simulink model "Minh_Final_project_Inverter_V3"  (R2024b)
settings: Solver=VariableStepAuto  StartTime=0.0  StopTime=100  FixedStep=1e-5  MaxStep=1e-3  MinStep=1e-8  RelTol=1e-2
values from neighbouring files (symbols this model uses):
  A_f = 1.24    [Minh_Inverter_Init.m]
  C_d = 0.7041    [Minh_Inverter_Init.m]
  C_rr = 0.02    [Minh_Inverter_Init.m]
  Current_max = min(InvCurr,mCurr)    [Minh_Inverter_Init.m]
  Encoder_Offset = (PhaseA_offset/ppair)*pi/180    (= -0.785398163397)    [Minh_Inverter_Init.m]
  g = 9.8    [Minh_Inverter_Init.m]
  J = mrot*r^2/k^2 + 0.0045    (= 0.8303048)    [Minh_Inverter_Init.m]
  k = 1    [Minh_Inverter_Init.m]
  lambda = 0.0375    [Minh_Inverter_Init.m]
  Ld = 0.1e-3    (= 0.0001)    [Minh_Inverter_Init.m]
  Lq = Ld    (= 0.0001)    [Minh_Inverter_Init.m]
  m = 1    [Minh_Inverter_Init.m]
  ppair = 4    [Minh_Inverter_Init.m]
  r = 0.4064/2    (= 0.2032)    [Minh_Inverter_Init.m]
  rho = 1.2    [Minh_Inverter_Init.m]
  Rs = (Rpp^2)/(Rpp*3)    (= 0.00433333333333)    [Minh_Inverter_Init.m]
  speed_max = rpm_max*2*pi/60    (= 523.598775598)    [Minh_Inverter_Init.m]
  Torque_max = Current_max*3*lambda*ppair/2    [Minh_Inverter_Init.m]
  Voltage_max = min(V_bat,mVolt)    [Minh_Inverter_Init.m]
undefined symbols (not defined in the file or in its folder): Down, Up
libraries: nesl_utility x27, fl_lib x23, slpidlib x12, ee_lib x11, spsabctodq0Lib x4, simulink x3, spsdq0toabcLib x2, eePwmGenerator x2, mcbresolverdecoderlib x1, eeResolverToDigitalConverter x1
(part 2 of 3)

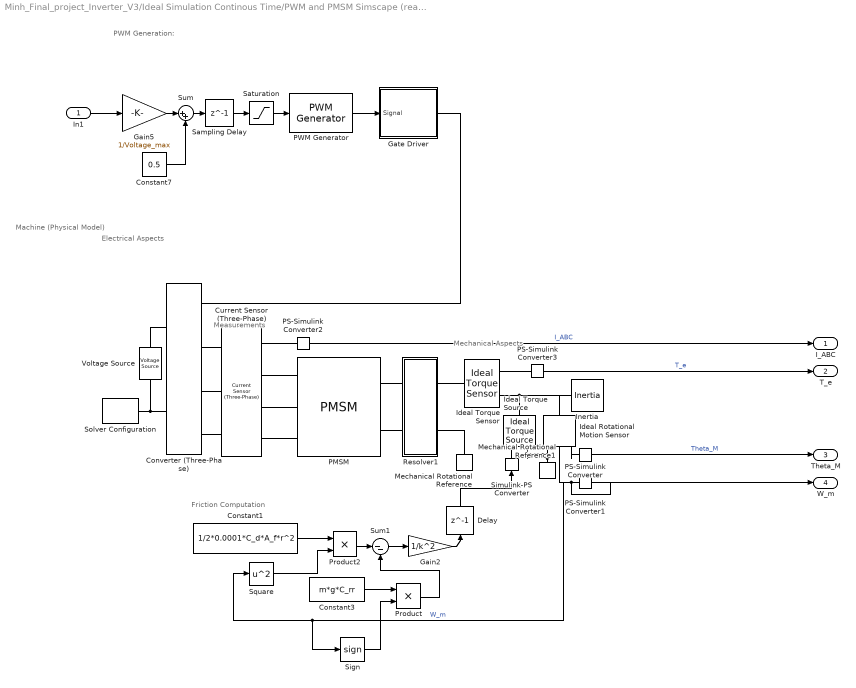
== system Minh_Final_project_Inverter_V3/Ideal Simulation Continous Time/PWM and PMSM Simscape (real model) ==
  note: Friction Computation
  note: Machine (Physical Model)
  note: Measurements
  note: Mechanical Aspects
  note: Electrical Aspects
  note: PWM Generation:
  In1 : Inport
  Constant1 : Constant  Value=1/2*0.0001*C_d*A_f*r^2
  Constant3 : Constant  Value=m*g*C_rr
  Constant7 : Constant  Value=0.5
  Converter (Three-Phase) : ee_lib/Semiconductors & Converters/Converters/Converter (Three-Phase)  port_option=ee.enum.threePhasePort.expanded  fidelity_option=ee.enum.converters.fidelity.detailed  device_type=ee.enum.converters.switchingdevice.ideal  showThermalPort=false  K=0  Vth=6 V  Vgt=1 V  Vgt_off=-1 V  Ih=1 A  Vf=0.8 V  Ron=0.001 Ohm  Rds=0.001 Ohm  Goff=1e-6 1/Ohm  Eon_scalar=22.86e-3 J  Eoff_scalar=17.14e-3 J  Eoff_natural_commutation=10e-3 J  Voff=300 V  Iout_scalar=600 A  onCurrentMeasDelay=0 s  useCurrentFromPreviousCycle=false  useVoltageFromPreviousCycle=false  diode_param=ee.enum.converters.protectiondiode.none  diode_Vf=0.8 V  diode_Ron=0.001 Ohm  diode_Goff=1e-5 1/Ohm  diode_C=50 nF  diode_iRM=-235 A  diode_iF=300 A  diode_idot=-50 A/us  diode_trr_param=ee.enum.converters.diodetrr.trr_factor  diode_trr_factor=3  diode_trr=15 us  diode_Qrr=1500 s*uA  diode_rec_loss_model=ee.enum.diode.reverseRecoveryModel.fixed  diode_ErecVal=0 J  diode_scaleWithIandV=false  diode_ErecMat=zeros(2, 3) J  diode_TjrecVec=[298.15, 398.15] K  diode_IfrecVec=[.1, 1, 10] A  diode_IrecVal=10 A  diode_VrecVal=10 V  diode_tFilter=1 / 1000 / 100 s  thermal_network_parameterization=ee.enum.thermalNetworkTopology.external  Rth=[.08, .5] K/W  Rth_Cauer=[.08, .1, .5] K/W  Rth_Foster=[.08, .14, .22, .16] K/W  thermal_mass_parameterization=ee.enum.thermalNetwork.timeconstant  thermal_mass=[.01, .5] J/K  thermal_mass_Cauer=[.01, .1, .5] J/K  thermal_mass_Foster=[.001, .005, .05, .5] J/K  thermal_time_constant=[.001, .2] s  thermal_time_constant_Cauer=[.001, .1, .2] s  thermal_time_constant_Foster=[7e-05, .0007, .01, .08] s  thermal_mass_initial_temperatures=[25, 25] degC  thermal_mass_initial_temperatures_Cauer=[25, 25, 25] degC  junction_thermal_mass=0.01 J/K  Tvec_initial_Foster=[25, 25, 25, 25] degC  snubber_type=ee.enum.converters.snubber.exclude  Cs=1e-7 F  Rs=0.1 Ohm  Vce_loss=[0, 150, 300] V
      settings: InternalSimscapePortConfiguration="{\"Bottom\":[],\"Left\":[{\"id\":\"G\",\"label\":\"G\",\"type\":\"foundation.electrical.twelve_phase\"},{\"id\":\"a\",\"label\":\"a\",\"type\":\"foundation.electrical.electrical\"},{\"id\":\"b\",\"label\":\"b\",\"type\":\"foundation.electrical.electrical\"},{\"id\":\"c\",\"label\":\"c\",\"type\":\"foundation.electrical.electrical\"}],\"Right\":[{\"id\":\"p\",\"label\":\"+\",\"type\":\"foundation.electrical.electrical\"},{\"id\":\"n\",\"label\":\"-\",\"type\":\"foundation.electrical.electrical\"}],\"Top\":[]}"
  Current Sensor (Three-Phase) : ee_lib/Sensors & Transducers/Current Sensor (Three-Phase)
      settings: InternalSimscapePortConfiguration="{\"Bottom\":[],\"Left\":[{\"id\":\"a1\",\"label\":\"a1\",\"type\":\"foundation.electrical.electrical\"},{\"id\":\"b1\",\"label\":\"b1\",\"type\":\"foundation.electrical.electrical\"},{\"id\":\"c1\",\"label\":\"c1\",\"type\":\"foundation.electrical.electrical\"}],\"Right\":[{\"id\":\"I_output\",\"label\":\"I\",\"type\":\"output\"},{\"id\":\"a2\",\"label\":\"a2\",\"type\":\"foundation.electrical.electrical\"},{\"id\":\"b2\",\"label\":\"b2\",\"type\":\"foundation.electrical.electrical\"},{\"id\":\"c2\",\"label\":\"c2\",\"type\":\"foundation.electrical.electrical\"}],\"Top\":[]}"
  Delay : Delay  DelayLength=1
  Gain2 : Gain  Gain=1/k^2
  Gain5 : Gain  Gain=1/Voltage_max
  Gate Driver : Subsystem
  Ideal Rotational Motion Sensor : fl_lib/Mechanical/Mechanical Sensors/Ideal Rotational Motion Sensor  reference=foundation.enum.MeasurementReference.difference  acceleration_port=false  velocity_port=true  position_port=true  wrap_angle=false  offset=0 rad
  Ideal Torque Sensor : fl_lib/Mechanical/Mechanical Sensors/Ideal Torque Sensor
  Ideal Torque Source : fl_lib/Mechanical/Mechanical Sources/Ideal Torque Source
  Inertia : fl_lib/Mechanical/Rotational Elements/Inertia  inertia=J kg*m^2  num_ports=foundation.enum.numPorts2.one  w_specify=off  w_priority=High  w=0 rad/s  w_nominal_specify=off  w_nominal_value=1  w_nominal_unit=rad/s  t_specify=off  t_priority=None  t=0 N*m  t_nominal_specify=off  t_nominal_value=1  t_nominal_unit=N*m
  Mechanical Rotational Reference : fl_lib/Mechanical/Rotational Elements/Mechanical Rotational Reference
  Mechanical Rotational Reference1 : fl_lib/Mechanical/Rotational Elements/Mechanical Rotational Reference
  PMSM : ee_lib/Electromechanical/Permanent Magnet/PMSM  port_option=ee.enum.threePhasePort.expanded  winding_type=ee.enum.statorconnection.wye  machine_param=ee.enum.pmsm.parameterization.constant  nPolePairs=ppair  pmflux_param=ee.enum.pmflux.fluxlinkage  pm_flux_linkage=lambda N*m/A  torque_constant=0.18 N*m/A  back_emf_constant=0.18 V*s/rad  stator_param=ee.enum.statorparam.LdLqL0  Ld=Ld H  Lq=Lq H  idVec=[-200, 0, 200] A  iqVec=[-200, 0, 200] A  LdMatrix=0.0002 * ones(3, 3) H  LqMatrix=0.0002 * ones(3, 3) H  PmMatrix=0.1 * ones(3, 3) Wb  ktMatrix=0.18 * ones(3, 3) N*m/A  keMatrix=0.18 * ones(3, 3) V*s/rad  L0=0.00016 H  Ls=0.0002 H  Lm=-0.00002 H  Ms=0.00002 H  Rs=Rs Ohm  zero_sequence=ee.enum.park.zerosequence.exclude  axes_param=ee.enum.rotorangle.daxis  loss_param=ee.enum.ironloss.none  losses_oc=[0, 0, 0] W  losses_sc=[0, 0, 0] W  f_losses=60 Hz  Isc_losses=95 A  J=0.000001 kg*m^2  lam=0 N*m*s/rad  i_d_specify=off  i_d_priority=None  i_d=0 A  i_d_nominal_specify=off  i_d_nominal_value=1  i_d_nominal_unit=A  i_q_specify=off  i_q_priority=None  i_q=0 A  i_q_nominal_specify=off  i_q_nominal_value=1  i_q_nominal_unit=A  torque_specify=off  torque_priority=None  torque=0 N*m  torque_nominal_specify=off  torque_nominal_value=1  torque_nominal_unit=N*m  angular_velocity_specify=off  angular_velocity_priority=High  angular_velocity=0 rpm  angular_velocity_nominal_specify=off  angular_velocity_nominal_value=1  angular_velocity_nominal_unit=rpm  angular_position_specify=off  angular_position_priority=High  angular_position=0 deg  angular_position_nominal_specify=off  angular_position_nominal_value=1  angular_position_nominal_unit=deg  alpha=3.93e-3 1/K  alpha_flux=-0.001 1/K  Tmeas=298.15 K  stator_thermal_mass=100 J/K  rotor_thermal_mass=200 J/K  Rm_percent_rotor=90  Rd_percent_rotor=30  temperatureA_specify=off  temperatureA_priority=High  temperatureA=25 degC  temperatureA_nominal_specify=off  temperatureA_nominal_value=1  temperatureA_nominal_unit=degC  temperatureB_specify=off  temperatureB_priority=High  temperatureB=25 degC  temperatureB_nominal_specify=off  temperatureB_nominal_value=1  temperatureB_nominal_unit=degC  temperatureC_specify=off  temperatureC_priority=High  temperatureC=25 degC  temperatureC_nominal_specify=off  temperatureC_nominal_value=1  temperatureC_nominal_unit=degC  temperatureR_specify=off  temperatureR_priority=High  temperatureR=25 degC  temperatureR_nominal_specify=off  temperatureR_nominal_value=1  temperatureR_nominal_unit=degC
      settings: InternalSimscapePortConfiguration="{\"Bottom\":[],\"Left\":[{\"id\":\"a\",\"label\":\"a\",\"type\":\"foundation.electrical.electrical\"},{\"id\":\"b\",\"label\":\"b\",\"type\":\"foundation.electrical.electrical\"},{\"id\":\"c\",\"label\":\"c\",\"type\":\"foundation.electrical.electrical\"}],\"Right\":[{\"id\":\"R\",\"label\":\"R\",\"type\":\"foundation.mechanical.rotational.rotational\"},{\"id\":\"C\",\"label\":\"C\",\"type\":\"foundation.mechanical.rotational.rotational\"}],\"Top\":[]}"
  PS-Simulink Converter{,1..3} (4 alike) : nesl_utility/PS-Simulink Converter  PhysicalDomain=network_engine_domain  SubClassName=ps_output  LeftPortType=input  RightPortType=output  PseudoPeriodic=off  Frequencies=[]  VectorFormat=inherit  Unit=inherit  AffineConversion=off
  PWM Generator : eePwmGenerator/PWM Generator  CarrCount=Up-Down  Tper=0.5/1e3  Tdelay=0  Ts=1e-6
  Product : Product
  Product2 : Product
  Resolver1 : Subsystem
  Sampling Delay : Delay  DelayLength=1  SampleTime=1e-6
  Saturation : Saturate  UpperLimit=1  LowerLimit=0
  Sign : Signum
  Simulink-PS Converter : nesl_utility/Simulink-PS Converter  PhysicalDomain=network_engine_domain  SubClassName=ps_input  LeftPortType=input  RightPortType=output  PseudoPeriodic=off  Frequencies=[]  NoiseDistribution=none  NoiseParameters=[]  Unit=1  AffineConversion=off  FilteringAndDerivatives=provide  SimscapeFilterOrder=1  InputFilterTimeConstant=0.001  UdotUserProvided=0
  Solver Configuration : nesl_utility/Solver Configuration  PhysicalDomain=network_engine_domain  SubClassName=solver  LeftPortType=input  RightPortType=generic  Tones=[]  Harmonics=[]  SimulateNoise=off  Profile=off  UseLocalSampling=off  EnableSwitchedLinearOptims=on  FrequencyDomain=off  UseCCode=off  RelTol=0.001  AbsTol=0.001  MinStep=1e-09  ToWorkspace=off  RevertToSquareIcSolve=off  NumHomotopyIterations=100  PhasorMode=off  PhasorModeNumHarmonics=1  ConsistencySolver=NEWTON_XTOL_AFTER_FTOL  IndexReductionMethod=None  DoDC=off  ResidualTolerance=1e-09  ConsistencyTolSource=GLOBAL  ConsistencyAbsTol=0.001  ConsistencyRelTol=0.001  ConsistencyTolFactor=0.001  UseLocalSolver=on  LocalSolverChoice=NE_TRAPEZOIDAL_ADVANCER  ResolveIndetEquations=on  FunctionEvalNumThread=1  LocalSolverSampleTime=1e-6  DoFixedCost=on  MaxNonlinIter=3  MaxModeIter=2  ComputeImpulses=off  ImpulseIterations=2  LinearAlgebra=auto  LinearAlgebraNumThread=0  EquationFormulation=NE_TIME_EF  DelaysMemoryBudget=1024  AutomaticFiltering=on  FilteringTimeConstant=0.001  PartitionStorageMethod=AS_NEEDED  PartitionMemoryBudget=1024  PartitionMethod=ROBUST  MultibodyUseLocalSolver=off  MultibodyLocalSolverChoice=ODE1  MultibodyLocalSolverSampleTime=0.001
  Square : Math  Operator=square
  Sum : Sum  Inputs=|++
  Sum1 : Sum  Inputs=|--
  Voltage Source : ee_lib/Sources/Voltage Source  dc_voltage=Voltage_max V  ac_voltage=0 V  ac_shift=0 rad  ac_frequency=60 Hz  noise_mode=ee.enum.sources.noise.Disabled  PSD=0 V^2/Hz  sample_time=1e-3 s  repeatability=ee.enum.sources.repeatability.NotRepeatable  user_seed=0  auto_seed=3499211588  i_specify=off  i_priority=None  i=0 A  i_nominal_specify=off  i_nominal_value=1  i_nominal_unit=A  v_specify=off  v_priority=None  v=0 V  v_nominal_specify=off  v_nominal_value=1  v_nominal_unit=V
  I_ABC : Outport
  T_e : Outport  Port=2
  Theta_M : Outport  Port=3
  W_m : Outport  Port=4
  wires:
  Delay/1 -> Simulink-PS Converter/1
  Saturation/1 -> PWM Generator/1
  PS-Simulink Converter1/1 -> Sign/1, Square/1, W_m/1  "W_m"
  PS-Simulink Converter/1 -> Theta_M/1  "Theta_M"
  PWM Generator/1 -> Gate Driver/1(Signal)
  Sum1/1 -> Gain2/1
  Square/1 -> Product2/2
  Constant7/1 -> Sum/2
  Gain5/1 -> Sum/1
  Sampling Delay/1 -> Saturation/1
  Product2/1 -> Sum1/1
  PS-Simulink Converter3/1 -> T_e/1  "T_e"
  Sum/1 -> Sampling Delay/1
  Gain2/1 -> Delay/1
  PS-Simulink Converter2/1 -> I_ABC/1  "I_ABC"
  Constant1/1 -> Product2/1
  In1/1 -> Gain5/1
  Sign/1 -> Product/2
  Product/1 -> Sum1/2
  Constant3/1 -> Product/1
  connections:
  PMSM/RConn2 -- Resolver1/LConn2
  Voltage Source/RConn1 -- Solver Configuration/RConn1 -- Converter (Three-Phase)/RConn2
  Simulink-PS Converter/RConn1 -- Ideal Torque Source/RConn1
  Converter (Three-Phase)/LConn2 -- Current Sensor (Three-Phase)/LConn1
  Current Sensor (Three-Phase)/RConn4 -- PMSM/LConn3
  Ideal Rotational Motion Sensor/RConn3 -- PS-Simulink Converter/LConn1
  Voltage Source/LConn1 -- Converter (Three-Phase)/RConn1
  Current Sensor (Three-Phase)/RConn3 -- PMSM/LConn2
  Converter (Three-Phase)/LConn3 -- Current Sensor (Three-Phase)/LConn2
  Current Sensor (Three-Phase)/RConn1 -- PS-Simulink Converter2/LConn1
  Ideal Rotational Motion Sensor/RConn1 -- Mechanical Rotational Reference1/LConn1 -- Ideal Torque Source/RConn2
  Ideal Torque Sensor/RConn2 -- PS-Simulink Converter3/LConn1
  PS-Simulink Converter1/LConn1 -- Ideal Rotational Motion Sensor/RConn2
  Ideal Torque Source/LConn1 -- Ideal Rotational Motion Sensor/LConn1 -- Inertia/LConn1 -- Ideal Torque Sensor/RConn1
  Gate Driver/RConn1 -- Converter (Three-Phase)/LConn1
  Converter (Three-Phase)/LConn4 -- Current Sensor (Three-Phase)/LConn3
  PMSM/LConn1 -- Current Sensor (Three-Phase)/RConn2
  Resolver1/LConn1 -- PMSM/RConn1
  Resolver1/RConn1 -- Ideal Torque Sensor/LConn1
  Resolver1/RConn2 -- Mechanical Rotational Reference/LConn1

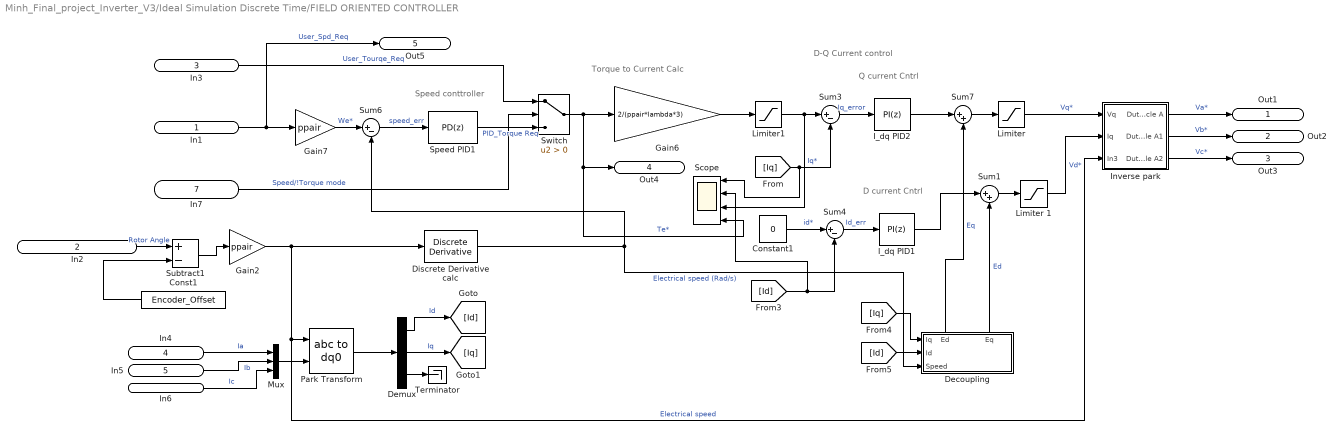
== system Minh_Final_project_Inverter_V3/Ideal Simulation Discrete Time/FIELD ORIENTED CONTROLLER ==
  note: Torque to Current Calc
  note: Speed conttroller
  note: D current
      | Cntrl
  note: D-Q Current control
  note: Q current
      | Cntrl
  In1 : Inport
  In2 : Inport  Port=2
  In3 : Inport  Port=3
  In4 : Inport  Port=4
  In5 : Inport  Port=5
  In6 : Inport  Port=6
  In7 : Inport  Port=7
  Const1 : Constant  Value=Encoder_Offset
  Constant1 : Constant  Value=0
  Decoupling : Subsystem
      settings: PortSchema="{\"entries\":[{\"content\":{\"sides\":[{\"content\":{\"connectorIds\":[\"In1\",\"In2\",\"In3\"]},\"type\":\"ConnectorPlacement.EquallySpacedRectSide\",\"uuid\":\"5f512ccb-8595-4499-a419-e995908cd1f5\"},{\"content\":{\"side\":\"RIGHT\"},\"type\":\"ConnectorPlacement.EquallySpacedRectSide\",\"uuid\":\"2a1de219-597a-4818-9587-d28590d7f25d\"},{\"content\":{\"connectorIds\":[\"Out1\",\"Out2\"],\"side\":\"TOP\"},\"type\":\"ConnectorPlacement.EquallySpacedRectSide\",\"uuid\":\"87b053a8-3806-4156-bae7-a97f33c02d51\"}]},\"type\":\"ConnectorPlacement.EquallySpacedConnector\",\"uuid\":\"5d9f8914-d3c5-4fbe-94a4-f1d2e0d8a5f7\"}],\"packageUris\":[\"http://schema.mathworks.com/mf0/Connector/R2020b\"],\"version\":\"1.0\"}"
  Demux : Demux  Outputs=3
  Discrete Derivative calc : simulink/Discrete/Discrete Derivative  gainval=1.0  ICPrevScaledInput=0.0  OutMin=[]  OutMax=[]  OutDataType=fixdt(1, 16)  OutScaling=2^-10  DoSatur=off
  Gain2 : Gain  Gain=ppair
  Gain6 : Gain  Gain=2/(ppair*lambda*3)
  Gain7 : Gain  Gain=ppair
  I_dq PID1 : slpidlib/PID Controller  Controller=PI  Form=Parallel  TimeDomain=Discrete-time  UseExternalTs=off  SampleTime=-1  IntegratorMethod=Forward Euler  FilterMethod=Forward Euler  ControllerParametersSource=internal  P=0.216674080570424  I=8.23559930371868  UseKiTs=off  D=2.81416629288768e-05  UseExternalDerivativeSource=off  N=4271.19819316481  UseFilter=on  TunerSelectOption=Transfer Function Based (PID Tuner App)  InitialConditionSource=internal  InitialConditionForIntegrator=0  InitialConditionForFilter=0  DifferentiatorICPrevScaledInput=0  ExternalReset=none  TrackingMode=off  Kt=1  LimitOutput=on  SatLimitsSource=internal  UpperSaturationLimit=Voltage_max  LowerSaturationLimit=-Voltage_max  LinearizeAsGain=off  AntiWindupMode=none  Kb=1  LimitIntegrator=on  UpperIntegratorSaturationLimit=Voltage_max  LowerIntegratorSaturationLimit=-Voltage_max  POutMin=[]  POutMax=[]  IOutMin=[]  IOutMax=[]  DOutMin=[]  DOutMax=[]  NOutMin=[]  NOutMax=[]  SumOutMin=[]  SumOutMax=[]  SaturationOutMin=[]  SaturationOutMax=[]  PParamMin=[]  PParamMax=[]  IParamMin=[]  IParamMax=[]  DParamMin=[]  DParamMax=[]  NParamMin=[]  NParamMax=[]  KbParamMin=[]  KbParamMax=[]  KtParamMin=[]  KtParamMax=[]  KbOutMin=[]  KbOutMax=[]  KtOutMin=[]  KtOutMax=[]  IntegratorOutMin=[]  IntegratorOutMax=[]  FilterOutMin=[]  FilterOutMax=[]  SumI1OutMin=[]  SumI1OutMax=[]  SumI2OutMin=[]  SumI2OutMax=[]  SumI3OutMin=[]  SumI3OutMax=[]  SumI4OutMin=[]  SumI4OutMax=[]  SumDOutMin=[]  SumDOutMax=[]  DifferentiatorOutMin=[]  DifferentiatorOutMax=[]  FilterDiffOutCoefMin=[]  FilterDiffOutCoefMax=[]  ReciprocalOutMin=[]  ReciprocalOutMax=[]  SumDenOutMin=[]  SumDenOutMax=[]  SumNumOutMin=[]  SumNumOutMax=[]  DivideOutMin=[]  DivideOutMax=[]  UdiffTsProdOutMin=[]  UdiffTsProdOutMax=[]  NTsProdOutMin=[]  NTsProdOutMax=[]  UintegralTsProdOutMin=[]  UintegralTsProdOutMax=[]  UngainTsProdOutMin=[]  UngainTsProdOutMax=[]  ClampingZeroOutDataTypeStr=Inherit: Inherit via back propagation  ClampingZeroOutMin=[]  ClampingZeroOutMax=[]  FilterDenConstantOutDataTypeStr=Inherit: Inherit via back propagation  FilterDenConstantOutMin=[]  FilterDenConstantOutMax=[]  PCopyOutDataTypeStr=Inherit: Inherit via back propagation  PCopyOutMin=[]  PCopyOutMax=[]  NCopyOutDataTypeStr=Inherit: Inherit via back propagation  NCopyOutMin=[]  NCopyOutMax=[]  IntegratorContinuousStateAttributes=''  IntegratorStateMustResolveToSignalObject=off  IntegratorRTWStateStorageClass=Auto  FilterContinuousStateAttributes=''  FilterStateMustResolveToSignalObject=off  FilterRTWStateStorageClass=Auto  ParallelPVariant=InternalParameters  IdealPVariant=Disabled  IVariant=InternalParameters  DVariant=Disabled  IntegratorVariant=Discrete  SatVariant=Enabled  AWVariant=Passthrough  PCopyVariant=Disabled  TRVariant=Disabled  FdbkBlocksVariant=Forward  IdealPFdbkVariant=Disabled  SatFdbkVariant=Disabled  DerivativeFilterVariant=Disabled  NVariant=Disabled  NCopyVariant=Disabled_SignalSpec  FilterICVariant=Disabled  IntegratorICVariant=InternalICs  ExternalResetVariant=Disabled  TRSumVariant=Passthrough  SumFdbkVariant=Disabled  SumVariant=Sum_PI  TsampFilterVariant=InternalTs  TsampNgainVariant=Passthrough  TsampIntegralVariant=Disabled_SignalSpec  ExternalSaturationOutDataTypeStr=Inherit: Same as second input  DerivativeSourceVariant=Disabled  PreIntVariant=InternalPreInt
  I_dq PID2 : slpidlib/PID Controller  Controller=PI  Form=Parallel  TimeDomain=Discrete-time  UseExternalTs=off  SampleTime=-1  IntegratorMethod=Forward Euler  FilterMethod=Forward Euler  ControllerParametersSource=internal  P=0.216674080570424  I=8.23559930371868  UseKiTs=off  D=2.81416629288768e-05  UseExternalDerivativeSource=off  N=4271.19819316481  UseFilter=on  TunerSelectOption=Transfer Function Based (PID Tuner App)  InitialConditionSource=internal  InitialConditionForIntegrator=0  InitialConditionForFilter=0  DifferentiatorICPrevScaledInput=0  ExternalReset=none  TrackingMode=off  Kt=1  LimitOutput=on  SatLimitsSource=internal  UpperSaturationLimit=Voltage_max  LowerSaturationLimit=-Voltage_max  LinearizeAsGain=off  AntiWindupMode=none  Kb=1  LimitIntegrator=on  UpperIntegratorSaturationLimit=Voltage_max  LowerIntegratorSaturationLimit=-Voltage_max  POutMin=[]  POutMax=[]  IOutMin=[]  IOutMax=[]  DOutMin=[]  DOutMax=[]  NOutMin=[]  NOutMax=[]  SumOutMin=[]  SumOutMax=[]  SaturationOutMin=[]  SaturationOutMax=[]  PParamMin=[]  PParamMax=[]  IParamMin=[]  IParamMax=[]  DParamMin=[]  DParamMax=[]  NParamMin=[]  NParamMax=[]  KbParamMin=[]  KbParamMax=[]  KtParamMin=[]  KtParamMax=[]  KbOutMin=[]  KbOutMax=[]  KtOutMin=[]  KtOutMax=[]  IntegratorOutMin=[]  IntegratorOutMax=[]  FilterOutMin=[]  FilterOutMax=[]  SumI1OutMin=[]  SumI1OutMax=[]  SumI2OutMin=[]  SumI2OutMax=[]  SumI3OutMin=[]  SumI3OutMax=[]  SumI4OutMin=[]  SumI4OutMax=[]  SumDOutMin=[]  SumDOutMax=[]  DifferentiatorOutMin=[]  DifferentiatorOutMax=[]  FilterDiffOutCoefMin=[]  FilterDiffOutCoefMax=[]  ReciprocalOutMin=[]  ReciprocalOutMax=[]  SumDenOutMin=[]  SumDenOutMax=[]  SumNumOutMin=[]  SumNumOutMax=[]  DivideOutMin=[]  DivideOutMax=[]  UdiffTsProdOutMin=[]  UdiffTsProdOutMax=[]  NTsProdOutMin=[]  NTsProdOutMax=[]  UintegralTsProdOutMin=[]  UintegralTsProdOutMax=[]  UngainTsProdOutMin=[]  UngainTsProdOutMax=[]  ClampingZeroOutDataTypeStr=Inherit: Inherit via back propagation  ClampingZeroOutMin=[]  ClampingZeroOutMax=[]  FilterDenConstantOutDataTypeStr=Inherit: Inherit via back propagation  FilterDenConstantOutMin=[]  FilterDenConstantOutMax=[]  PCopyOutDataTypeStr=Inherit: Inherit via back propagation  PCopyOutMin=[]  PCopyOutMax=[]  NCopyOutDataTypeStr=Inherit: Inherit via back propagation  NCopyOutMin=[]  NCopyOutMax=[]  IntegratorContinuousStateAttributes=''  IntegratorStateMustResolveToSignalObject=off  IntegratorRTWStateStorageClass=Auto  FilterContinuousStateAttributes=''  FilterStateMustResolveToSignalObject=off  FilterRTWStateStorageClass=Auto  ParallelPVariant=InternalParameters  IdealPVariant=Disabled  IVariant=InternalParameters  DVariant=Disabled  IntegratorVariant=Discrete  SatVariant=Enabled  AWVariant=Passthrough  PCopyVariant=Disabled  TRVariant=Disabled  FdbkBlocksVariant=Forward  IdealPFdbkVariant=Disabled  SatFdbkVariant=Disabled  DerivativeFilterVariant=Disabled  NVariant=Disabled  NCopyVariant=Disabled_SignalSpec  FilterICVariant=Disabled  IntegratorICVariant=InternalICs  ExternalResetVariant=Disabled  TRSumVariant=Passthrough  SumFdbkVariant=Disabled  SumVariant=Sum_PI  TsampFilterVariant=InternalTs  TsampNgainVariant=Passthrough  TsampIntegralVariant=Disabled_SignalSpec  ExternalSaturationOutDataTypeStr=Inherit: Same as second input  DerivativeSourceVariant=Disabled  PreIntVariant=InternalPreInt
  Inverse park : Subsystem
  Limiter : Saturate  UpperLimit=Voltage_max  LowerLimit=0  LinearizeAsGain=off
  Limiter 1 : Saturate  UpperLimit=Voltage_max  LowerLimit=0  LinearizeAsGain=off
  Limiter1 : Saturate  UpperLimit=Current_max  LowerLimit=-Current_max  LinearizeAsGain=off
  Mux : Mux  Inputs=3
  Park Transform : spsabctodq0Lib/abc to dq0  Alignment=Aligned with phase A axis
  Scope : Scope  NumInputPorts=4
  Speed PID1 : slpidlib/PID Controller  Controller=PD  Form=Parallel  TimeDomain=Discrete-time  UseExternalTs=off  SampleTime=-1  IntegratorMethod=Forward Euler  FilterMethod=Forward Euler  ControllerParametersSource=internal  P=20.6545195236646  I=640.266262711417  UseKiTs=off  D=0.00205517598679868  UseExternalDerivativeSource=off  N=100.498329175013  UseFilter=on  TunerSelectOption=Transfer Function Based (PID Tuner App)  InitialConditionSource=internal  InitialConditionForIntegrator=0  InitialConditionForFilter=0  DifferentiatorICPrevScaledInput=0  ExternalReset=none  TrackingMode=off  Kt=1  LimitOutput=on  SatLimitsSource=internal  UpperSaturationLimit=Torque_max  LowerSaturationLimit=-Torque_max  LinearizeAsGain=off  AntiWindupMode=none  Kb=1  LimitIntegrator=on  UpperIntegratorSaturationLimit=Torque_max  LowerIntegratorSaturationLimit=-Torque_max  RndMeth=Nearest  POutMin=[]  POutMax=[]  IOutMin=[]  IOutMax=[]  DOutMin=[]  DOutMax=[]  NOutMin=[]  NOutMax=[]  SumOutMin=[]  SumOutMax=[]  SaturationOutMin=[]  SaturationOutMax=[]  PParamMin=[]  PParamMax=[]  IParamMin=[]  IParamMax=[]  DParamMin=[]  DParamMax=[]  NParamMin=[]  NParamMax=[]  KbParamMin=[]  KbParamMax=[]  KtParamMin=[]  KtParamMax=[]  KbOutMin=[]  KbOutMax=[]  KtOutMin=[]  KtOutMax=[]  IntegratorOutMin=[]  IntegratorOutMax=[]  FilterOutMin=[]  FilterOutMax=[]  SumI1OutMin=[]  SumI1OutMax=[]  SumI2OutMin=[]  SumI2OutMax=[]  SumI3OutMin=[]  SumI3OutMax=[]  SumI4OutMin=[]  SumI4OutMax=[]  SumDOutMin=[]  SumDOutMax=[]  DifferentiatorOutMin=[]  DifferentiatorOutMax=[]  FilterDiffOutCoefMin=[]  FilterDiffOutCoefMax=[]  ReciprocalOutMin=[]  ReciprocalOutMax=[]  SumDenOutMin=[]  SumDenOutMax=[]  SumNumOutMin=[]  SumNumOutMax=[]  DivideOutMin=[]  DivideOutMax=[]  UdiffTsProdOutMin=[]  UdiffTsProdOutMax=[]  NTsProdOutMin=[]  NTsProdOutMax=[]  UintegralTsProdOutMin=[]  UintegralTsProdOutMax=[]  UngainTsProdOutMin=[]  UngainTsProdOutMax=[]  ClampingZeroOutDataTypeStr=Inherit: Inherit via back propagation  ClampingZeroOutMin=[]  ClampingZeroOutMax=[]  FilterDenConstantOutDataTypeStr=Inherit: Inherit via back propagation  FilterDenConstantOutMin=[]  FilterDenConstantOutMax=[]  PCopyOutDataTypeStr=Inherit: Inherit via back propagation  PCopyOutMin=[]  PCopyOutMax=[]  NCopyOutDataTypeStr=Inherit: Inherit via back propagation  NCopyOutMin=[]  NCopyOutMax=[]  IntegratorContinuousStateAttributes=''  IntegratorStateMustResolveToSignalObject=off  IntegratorRTWStateStorageClass=Auto  FilterContinuousStateAttributes=''  FilterStateMustResolveToSignalObject=off  FilterRTWStateStorageClass=Auto  ParallelPVariant=InternalParameters  IdealPVariant=Disabled  IVariant=Disabled  DVariant=InternalParameters  IntegratorVariant=Disabled  SatVariant=Enabled  AWVariant=Disabled  PCopyVariant=Disabled  TRVariant=Disabled  FdbkBlocksVariant=Forward  IdealPFdbkVariant=Disabled  SatFdbkVariant=Disabled  DerivativeFilterVariant=ForwardEulerFilter  NVariant=InternalParameters  NCopyVariant=Disabled  FilterICVariant=InternalICsFilter  IntegratorICVariant=Disabled  ExternalResetVariant=Disabled  TRSumVariant=Passthrough  SumFdbkVariant=Disabled  SumVariant=Sum_PD  TsampFilterVariant=InternalTs  TsampNgainVariant=Passthrough  TsampIntegralVariant=Disabled_SignalSpec  ExternalSaturationOutDataTypeStr=Inherit: Same as second input  DerivativeSourceVariant=ErrorSignal  PreIntVariant=InternalPreInt
  Subtract1 : Sum  Inputs=+-
  Sum1 : Sum  Inputs=|++
  Sum3 : Sum  Inputs=|+-
  Sum4 : Sum  Inputs=|+-
  Sum6 : Sum  Inputs=|+-
  Sum7 : Sum  Inputs=|++
  Switch : Switch  Criteria=u2 > Threshold  SaturateOnIntegerOverflow=off  InputSameDT=off
  Terminator : Terminator
  Out1 : Outport
  Out2 : Outport  Port=2
  Out3 : Outport  Port=3
  Out4 : Outport  Port=4
  Out5 : Outport  Port=5
  wires:
  In5/1 -> Mux/2  "Ib"
  In6/1 -> Mux/3  "Ic"
  Discrete Derivative calc/1 -> Sum6/2, Decoupling/3(Speed)  "Electrical speed (Rad/s)"
  I_dq PID1/1 -> Sum1/1
  [Id] -> Scope/2, Sum4/2
  Demux/2 -> [Iq]  "Iq"
  Inverse park/1(Duty Cycle A) -> Out1/1  "Va*"
  I_dq PID2/1 -> Sum7/1
  Inverse park/3(Duty Cycle A2) -> Out3/1  "Vc*"
  [Iq] -> Scope/1, Sum3/2
  Switch/1 -> Scope/4, Out4/1, Gain6/1  "Te*"
  Demux/1 -> [Id]  "Id"
  [Iq] -> Decoupling/1(Iq)
  Demux/3 -> Terminator/1
  Sum3/1 -> I_dq PID2/1  "Iq_error"
  Decoupling/2(Eq) -> Sum1/2  "Ed"
  Sum7/1 -> Limiter/1
  Limiter 1/1 -> Inverse park/2(Iq)  "Vd*"
  Decoupling/1(Ed) -> Sum7/2  "Eq"
  In1/1 -> Out5/1, Gain7/1  "User_Spd_Req"
  Inverse park/2(Duty Cycle A1) -> Out2/1  "Vb*"
  Sum4/1 -> I_dq PID1/1  "Id_err"
  Sum1/1 -> Limiter 1/1
  Sum6/1 -> Speed PID1/1  "speed_err"
  Constant1/1 -> Sum4/1  "id*"
  Speed PID1/1 -> Switch/3  "PID_Torque Req"
  [Id] -> Decoupling/2(Id)
  In4/1 -> Mux/1  "Ia"
  Limiter/1 -> Inverse park/1(Vq)  "Vq*"
  Mux/1 -> Park Transform/1
  Gain6/1 -> Limiter1/1
  In3/1 -> Switch/1  "User_Tourqe_Req"
  Park Transform/1 -> Demux/1
  In7/1 -> Switch/2  "Speed/!Torque mode"
  Limiter1/1 -> Scope/3, Sum3/1  "Iq*"
  Gain7/1 -> Sum6/1  "We*"
  Gain2/1 -> Discrete Derivative calc/1, Park Transform/2, Inverse park/3(In3)  "Electrical speed"
  Const1/1 -> Subtract1/2
  Subtract1/1 -> Gain2/1
  In2/1 -> Subtract1/1  "Rotor Angle"

== system Minh_Final_project_Inverter_V3/Ideal Simulation Discrete Time/PMSM Mathematical model ==
  note: PMSM (Mathematical Model)
  abc : Inport
  Constant3 : Constant  Value=0
  Demux1 : Demux  Outputs=3
  Gain6 : Gain  Gain=1/ppair
  Machine Model in DQ : Subsystem
  Mechanical Model : Subsystem
  Mux1 : Mux  Inputs=3
  Terminator : Terminator
  abc to dq0 : spsabctodq0Lib/abc to dq0  Alignment=Aligned with phase A axis
  dq0 to abc : spsdq0toabcLib/dq0 to abc  Alignment=Aligned with phase A axis
  abc1 : Outport
  Out3 : Outport  Port=2
  T_e : Outport  Port=3
  w_m : Outport  Port=4
  wires:
  Demux1/2 -> Machine Model in DQ/2(v_q)
  Machine Model in DQ/3(th_e) -> abc to dq0/2, dq0 to abc/2, Gain6/1
  Demux1/1 -> Machine Model in DQ/1(v_d)
  Mux1/1 -> dq0 to abc/1
  Mechanical Model/1(w_m) -> w_m/1, Machine Model in DQ/3(w_m)
  Machine Model in DQ/4(T_e) -> T_e/1, Mechanical Model/1(T_e)  "Tourqe"
  Constant3/1 -> Mux1/3
  Demux1/3 -> Terminator/1
  Machine Model in DQ/1(i_d) -> Mux1/1  "i_d"
  Machine Model in DQ/2(i_q) -> Mux1/2  "i_q"
  abc to dq0/1 -> Demux1/1
  dq0 to abc/1 -> abc1/1
  abc/1 -> abc to dq0/1
  Gain6/1 -> Out3/1  "Rotor Angle"

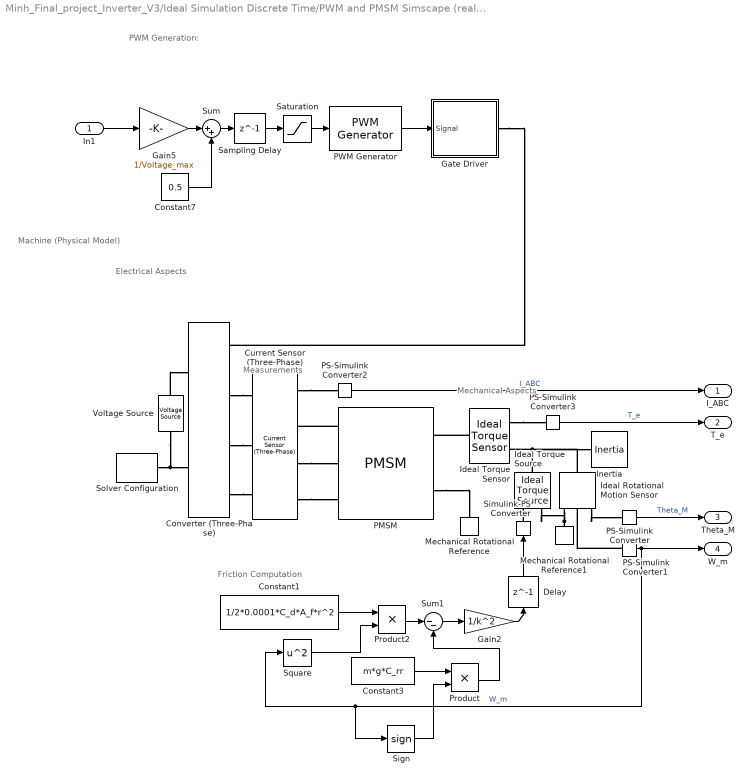
== system Minh_Final_project_Inverter_V3/Ideal Simulation Discrete Time/PWM and PMSM Simscape (real model) ==
  note: Friction Computation
  note: Machine (Physical Model)
  note: Measurements
  note: Mechanical Aspects
  note: Electrical Aspects
  note: PWM Generation:
  In1 : Inport
  Constant1 : Constant  Value=1/2*0.0001*C_d*A_f*r^2
  Constant3 : Constant  Value=m*g*C_rr
  Constant7 : Constant  Value=0.5
  Converter (Three-Phase) : ee_lib/Semiconductors & Converters/Converters/Converter (Three-Phase)  port_option=ee.enum.threePhasePort.expanded  fidelity_option=ee.enum.converters.fidelity.detailed  device_type=ee.enum.converters.switchingdevice.ideal  showThermalPort=false  K=0  Vth=6 V  Vgt=1 V  Vgt_off=-1 V  Ih=1 A  Vf=0.8 V  Ron=0.001 Ohm  Rds=0.001 Ohm  Goff=1e-6 1/Ohm  Eon_scalar=22.86e-3 J  Eoff_scalar=17.14e-3 J  Eoff_natural_commutation=10e-3 J  Voff=300 V  Iout_scalar=600 A  onCurrentMeasDelay=0 s  useCurrentFromPreviousCycle=false  useVoltageFromPreviousCycle=false  diode_param=ee.enum.converters.protectiondiode.none  diode_Vf=0.8 V  diode_Ron=0.001 Ohm  diode_Goff=1e-5 1/Ohm  diode_C=50 nF  diode_iRM=-235 A  diode_iF=300 A  diode_idot=-50 A/us  diode_trr_param=ee.enum.converters.diodetrr.trr_factor  diode_trr_factor=3  diode_trr=15 us  diode_Qrr=1500 s*uA  diode_rec_loss_model=ee.enum.diode.reverseRecoveryModel.fixed  diode_ErecVal=0 J  diode_scaleWithIandV=false  diode_ErecMat=zeros(2, 3) J  diode_TjrecVec=[298.15, 398.15] K  diode_IfrecVec=[.1, 1, 10] A  diode_IrecVal=10 A  diode_VrecVal=10 V  diode_tFilter=1 / 1000 / 100 s  thermal_network_parameterization=ee.enum.thermalNetworkTopology.external  Rth=[.08, .5] K/W  Rth_Cauer=[.08, .1, .5] K/W  Rth_Foster=[.08, .14, .22, .16] K/W  thermal_mass_parameterization=ee.enum.thermalNetwork.timeconstant  thermal_mass=[.01, .5] J/K  thermal_mass_Cauer=[.01, .1, .5] J/K  thermal_mass_Foster=[.001, .005, .05, .5] J/K  thermal_time_constant=[.001, .2] s  thermal_time_constant_Cauer=[.001, .1, .2] s  thermal_time_constant_Foster=[7e-05, .0007, .01, .08] s  thermal_mass_initial_temperatures=[25, 25] degC  thermal_mass_initial_temperatures_Cauer=[25, 25, 25] degC  junction_thermal_mass=0.01 J/K  Tvec_initial_Foster=[25, 25, 25, 25] degC  snubber_type=ee.enum.converters.snubber.exclude  Cs=1e-7 F  Rs=0.1 Ohm  Vce_loss=[0, 150, 300] V
      settings: InternalSimscapePortConfiguration="{\"Bottom\":[],\"Left\":[{\"id\":\"G\",\"label\":\"G\",\"type\":\"foundation.electrical.twelve_phase\"},{\"id\":\"a\",\"label\":\"a\",\"type\":\"foundation.electrical.electrical\"},{\"id\":\"b\",\"label\":\"b\",\"type\":\"foundation.electrical.electrical\"},{\"id\":\"c\",\"label\":\"c\",\"type\":\"foundation.electrical.electrical\"}],\"Right\":[{\"id\":\"p\",\"label\":\"+\",\"type\":\"foundation.electrical.electrical\"},{\"id\":\"n\",\"label\":\"-\",\"type\":\"foundation.electrical.electrical\"}],\"Top\":[]}"
  Current Sensor (Three-Phase) : ee_lib/Sensors & Transducers/Current Sensor (Three-Phase)
      settings: InternalSimscapePortConfiguration="{\"Bottom\":[],\"Left\":[{\"id\":\"a1\",\"label\":\"a1\",\"type\":\"foundation.electrical.electrical\"},{\"id\":\"b1\",\"label\":\"b1\",\"type\":\"foundation.electrical.electrical\"},{\"id\":\"c1\",\"label\":\"c1\",\"type\":\"foundation.electrical.electrical\"}],\"Right\":[{\"id\":\"I_output\",\"label\":\"I\",\"type\":\"output\"},{\"id\":\"a2\",\"label\":\"a2\",\"type\":\"foundation.electrical.electrical\"},{\"id\":\"b2\",\"label\":\"b2\",\"type\":\"foundation.electrical.electrical\"},{\"id\":\"c2\",\"label\":\"c2\",\"type\":\"foundation.electrical.electrical\"}],\"Top\":[]}"
  Delay : Delay  DelayLength=1
  Gain2 : Gain  Gain=1/k^2
  Gain5 : Gain  Gain=1/Voltage_max
  Gate Driver : Subsystem
  Ideal Rotational Motion Sensor : fl_lib/Mechanical/Mechanical Sensors/Ideal Rotational Motion Sensor  reference=foundation.enum.MeasurementReference.difference  acceleration_port=false  velocity_port=true  position_port=true  wrap_angle=false  offset=0 rad
  Ideal Torque Sensor : fl_lib/Mechanical/Mechanical Sensors/Ideal Torque Sensor
  Ideal Torque Source : fl_lib/Mechanical/Mechanical Sources/Ideal Torque Source
  Inertia : fl_lib/Mechanical/Rotational Elements/Inertia  inertia=J kg*m^2  num_ports=foundation.enum.numPorts2.one  w_specify=off  w_priority=High  w=0 rad/s  w_nominal_specify=off  w_nominal_value=1  w_nominal_unit=rad/s  t_specify=off  t_priority=None  t=0 N*m  t_nominal_specify=off  t_nominal_value=1  t_nominal_unit=N*m
  Mechanical Rotational Reference : fl_lib/Mechanical/Rotational Elements/Mechanical Rotational Reference
  Mechanical Rotational Reference1 : fl_lib/Mechanical/Rotational Elements/Mechanical Rotational Reference
  PMSM : ee_lib/Electromechanical/Permanent Magnet/PMSM  port_option=ee.enum.threePhasePort.expanded  winding_type=ee.enum.statorconnection.wye  machine_param=ee.enum.pmsm.parameterization.constant  nPolePairs=ppair  pmflux_param=ee.enum.pmflux.fluxlinkage  pm_flux_linkage=lambda N*m/A  torque_constant=0.18 N*m/A  back_emf_constant=0.18 V*s/rad  stator_param=ee.enum.statorparam.LdLqL0  Ld=Ld H  Lq=Lq H  idVec=[-200, 0, 200] A  iqVec=[-200, 0, 200] A  LdMatrix=0.0002 * ones(3, 3) H  LqMatrix=0.0002 * ones(3, 3) H  PmMatrix=0.1 * ones(3, 3) Wb  ktMatrix=0.18 * ones(3, 3) N*m/A  keMatrix=0.18 * ones(3, 3) V*s/rad  L0=0.00016 H  Ls=0.0002 H  Lm=-0.00002 H  Ms=0.00002 H  Rs=Rs Ohm  zero_sequence=ee.enum.park.zerosequence.exclude  axes_param=ee.enum.rotorangle.daxis  loss_param=ee.enum.ironloss.none  losses_oc=[0, 0, 0] W  losses_sc=[0, 0, 0] W  f_losses=60 Hz  Isc_losses=95 A  J=0.000001 kg*m^2  lam=0 N*m*s/rad  i_d_specify=off  i_d_priority=None  i_d=0 A  i_d_nominal_specify=off  i_d_nominal_value=1  i_d_nominal_unit=A  i_q_specify=off  i_q_priority=None  i_q=0 A  i_q_nominal_specify=off  i_q_nominal_value=1  i_q_nominal_unit=A  torque_specify=off  torque_priority=None  torque=0 N*m  torque_nominal_specify=off  torque_nominal_value=1  torque_nominal_unit=N*m  angular_velocity_specify=off  angular_velocity_priority=High  angular_velocity=0 rpm  angular_velocity_nominal_specify=off  angular_velocity_nominal_value=1  angular_velocity_nominal_unit=rpm  angular_position_specify=off  angular_position_priority=High  angular_position=0 deg  angular_position_nominal_specify=off  angular_position_nominal_value=1  angular_position_nominal_unit=deg  alpha=3.93e-3 1/K  alpha_flux=-0.001 1/K  Tmeas=298.15 K  stator_thermal_mass=100 J/K  rotor_thermal_mass=200 J/K  Rm_percent_rotor=90  Rd_percent_rotor=30  temperatureA_specify=off  temperatureA_priority=High  temperatureA=25 degC  temperatureA_nominal_specify=off  temperatureA_nominal_value=1  temperatureA_nominal_unit=degC  temperatureB_specify=off  temperatureB_priority=High  temperatureB=25 degC  temperatureB_nominal_specify=off  temperatureB_nominal_value=1  temperatureB_nominal_unit=degC  temperatureC_specify=off  temperatureC_priority=High  temperatureC=25 degC  temperatureC_nominal_specify=off  temperatureC_nominal_value=1  temperatureC_nominal_unit=degC  temperatureR_specify=off  temperatureR_priority=High  temperatureR=25 degC  temperatureR_nominal_specify=off  temperatureR_nominal_value=1  temperatureR_nominal_unit=degC
      settings: InternalSimscapePortConfiguration="{\"Bottom\":[],\"Left\":[{\"id\":\"a\",\"label\":\"a\",\"type\":\"foundation.electrical.electrical\"},{\"id\":\"b\",\"label\":\"b\",\"type\":\"foundation.electrical.electrical\"},{\"id\":\"c\",\"label\":\"c\",\"type\":\"foundation.electrical.electrical\"}],\"Right\":[{\"id\":\"R\",\"label\":\"R\",\"type\":\"foundation.mechanical.rotational.rotational\"},{\"id\":\"C\",\"label\":\"C\",\"type\":\"foundation.mechanical.rotational.rotational\"}],\"Top\":[]}"
  PS-Simulink Converter{,1..3} (4 alike) : nesl_utility/PS-Simulink Converter  PhysicalDomain=network_engine_domain  SubClassName=ps_output  LeftPortType=input  RightPortType=output  PseudoPeriodic=off  Frequencies=[]  VectorFormat=inherit  Unit=inherit  AffineConversion=off
  PWM Generator : eePwmGenerator/PWM Generator  CarrCount=Up-Down  Tper=0.5/1e3  Tdelay=0  Ts=1e-6
  Product : Product
  Product2 : Product
  Sampling Delay : Delay  DelayLength=1  SampleTime=1e-6
  Saturation : Saturate  UpperLimit=1  LowerLimit=0
  Sign : Signum
  Simulink-PS Converter : nesl_utility/Simulink-PS Converter  PhysicalDomain=network_engine_domain  SubClassName=ps_input  LeftPortType=input  RightPortType=output  PseudoPeriodic=off  Frequencies=[]  NoiseDistribution=none  NoiseParameters=[]  Unit=1  AffineConversion=off  FilteringAndDerivatives=provide  SimscapeFilterOrder=1  InputFilterTimeConstant=0.001  UdotUserProvided=0
  Solver Configuration : nesl_utility/Solver Configuration  PhysicalDomain=network_engine_domain  SubClassName=solver  LeftPortType=input  RightPortType=generic  Tones=[]  Harmonics=[]  SimulateNoise=off  Profile=off  UseLocalSampling=off  EnableSwitchedLinearOptims=on  FrequencyDomain=off  UseCCode=off  RelTol=0.001  AbsTol=0.001  MinStep=1e-09  ToWorkspace=off  RevertToSquareIcSolve=off  NumHomotopyIterations=100  PhasorMode=off  PhasorModeNumHarmonics=1  ConsistencySolver=NEWTON_XTOL_AFTER_FTOL  IndexReductionMethod=None  DoDC=off  ResidualTolerance=1e-09  ConsistencyTolSource=GLOBAL  ConsistencyAbsTol=0.001  ConsistencyRelTol=0.001  ConsistencyTolFactor=0.001  UseLocalSolver=on  LocalSolverChoice=NE_TRAPEZOIDAL_ADVANCER  ResolveIndetEquations=on  FunctionEvalNumThread=1  LocalSolverSampleTime=1e-6  DoFixedCost=on  MaxNonlinIter=3  MaxModeIter=2  ComputeImpulses=off  ImpulseIterations=2  LinearAlgebra=auto  LinearAlgebraNumThread=0  EquationFormulation=NE_TIME_EF  DelaysMemoryBudget=1024  AutomaticFiltering=on  FilteringTimeConstant=0.001  PartitionStorageMethod=AS_NEEDED  PartitionMemoryBudget=1024  PartitionMethod=ROBUST  MultibodyUseLocalSolver=off  MultibodyLocalSolverChoice=ODE1  MultibodyLocalSolverSampleTime=0.001
  Square : Math  Operator=square
  Sum : Sum  Inputs=|++
  Sum1 : Sum  Inputs=|--
  Voltage Source : ee_lib/Sources/Voltage Source  dc_voltage=Voltage_max V  ac_voltage=0 V  ac_shift=0 rad  ac_frequency=60 Hz  noise_mode=ee.enum.sources.noise.Disabled  PSD=0 V^2/Hz  sample_time=1e-3 s  repeatability=ee.enum.sources.repeatability.NotRepeatable  user_seed=0  auto_seed=3922919431  i_specify=off  i_priority=None  i=0 A  i_nominal_specify=off  i_nominal_value=1  i_nominal_unit=A  v_specify=off  v_priority=None  v=0 V  v_nominal_specify=off  v_nominal_value=1  v_nominal_unit=V
  I_ABC : Outport
  T_e : Outport  Port=2
  Theta_M : Outport  Port=3
  W_m : Outport  Port=4
  wires:
  Delay/1 -> Simulink-PS Converter/1
  Saturation/1 -> PWM Generator/1
  PS-Simulink Converter1/1 -> W_m/1, Sign/1, Square/1  "W_m"
  PS-Simulink Converter/1 -> Theta_M/1  "Theta_M"
  PWM Generator/1 -> Gate Driver/1(Signal)
  Sum1/1 -> Gain2/1
  Square/1 -> Product2/2
  Constant7/1 -> Sum/2
  Gain5/1 -> Sum/1
  Sampling Delay/1 -> Saturation/1
  Product2/1 -> Sum1/1
  PS-Simulink Converter3/1 -> T_e/1  "T_e"
  Sum/1 -> Sampling Delay/1
  Gain2/1 -> Delay/1
  PS-Simulink Converter2/1 -> I_ABC/1  "I_ABC"
  Constant1/1 -> Product2/1
  In1/1 -> Gain5/1
  Sign/1 -> Product/2
  Product/1 -> Sum1/2
  Constant3/1 -> Product/1
  connections:
  PMSM/RConn2 -- Mechanical Rotational Reference/LConn1
  Voltage Source/RConn1 -- Solver Configuration/RConn1 -- Converter (Three-Phase)/RConn2
  Simulink-PS Converter/RConn1 -- Ideal Torque Source/RConn1
  Converter (Three-Phase)/LConn2 -- Current Sensor (Three-Phase)/LConn1
  Current Sensor (Three-Phase)/RConn4 -- PMSM/LConn3
  Ideal Rotational Motion Sensor/RConn3 -- PS-Simulink Converter/LConn1
  Voltage Source/LConn1 -- Converter (Three-Phase)/RConn1
  Current Sensor (Three-Phase)/RConn3 -- PMSM/LConn2
  Converter (Three-Phase)/LConn3 -- Current Sensor (Three-Phase)/LConn2
  Current Sensor (Three-Phase)/RConn1 -- PS-Simulink Converter2/LConn1
  Ideal Rotational Motion Sensor/RConn1 -- Mechanical Rotational Reference1/LConn1 -- Ideal Torque Source/RConn2
  Ideal Torque Sensor/RConn2 -- PS-Simulink Converter3/LConn1
  PS-Simulink Converter1/LConn1 -- Ideal Rotational Motion Sensor/RConn2
  Ideal Torque Source/LConn1 -- Ideal Rotational Motion Sensor/LConn1 -- Inertia/LConn1 -- Ideal Torque Sensor/RConn1
  Gate Driver/RConn1 -- Converter (Three-Phase)/LConn1
  Converter (Three-Phase)/LConn4 -- Current Sensor (Three-Phase)/LConn3
  PMSM/LConn1 -- Current Sensor (Three-Phase)/RConn2
  Ideal Torque Sensor/LConn1 -- PMSM/RConn1

== system Minh_Final_project_Inverter_V3/Speed Controller Tuning/Mechanical Model ==
  T_e : Inport
  Constant1 : Constant  Value=1/2*rho*C_d*A_f*r^2
  Gain : Gain  Gain=1/k^2
  Product2 : Product
  Square : Math  Operator=square
  Subtract : Sum  Inputs=|+-
  Transfer Fcn : TransferFcn  Denominator=[J 0]
  w_m : Outport
  wires:
  Constant1/1 -> Product2/1
  Transfer Fcn/1 -> Square/1, w_m/1
  Product2/1 -> Gain/1
  Square/1 -> Product2/2
  Subtract/1 -> Transfer Fcn/1
  T_e/1 -> Subtract/1
  Gain/1 -> Subtract/2

== system Minh_Final_project_Inverter_V3/Ideal Simulation Continous Time/FIELD ORIENTED CONTROLLER/Decoupling ==
  Iq : Inport
  Id : Inport  Port=2
  Speed : Inport  Port=3
  Add1 : Sum
  Gain1 : Gain  Gain=-Lq
  Gain3 : Gain  Gain=Ld
  Gain4 : Gain  Gain=lambda
  Product : Product
  Product1 : Product
  Ed : Outport
  Eq : Outport  Port=2
  wires:
  Product/1 -> Ed/1
  Gain3/1 -> Product1/1
  Product1/1 -> Add1/1
  Gain4/1 -> Add1/2
  Add1/1 -> Eq/1
  Speed/1 -> Gain4/1, Gain3/1, Gain1/1  "Electrical Speed w_e"
  Iq/1 -> Product/1
  Gain1/1 -> Product/2
  Id/1 -> Product1/2

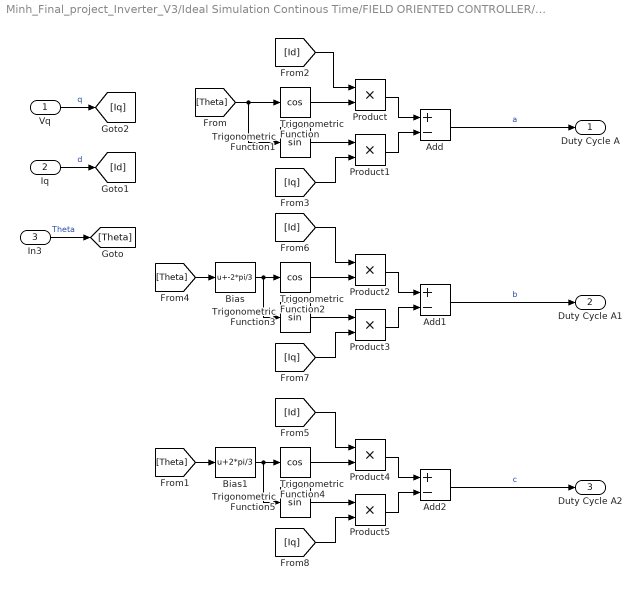
== system Minh_Final_project_Inverter_V3/Ideal Simulation Continous Time/FIELD ORIENTED CONTROLLER/Inverse park ==
  Vq : Inport
  Iq : Inport  Port=2
  In3 : Inport  Port=3
  Add : Sum  Inputs=+-
  Add1 : Sum  Inputs=+-
  Add2 : Sum  Inputs=+-
  Bias : Bias  Bias=-2*pi/3  SaturateOnIntegerOverflow=off
  Bias1 : Bias  Bias=2*pi/3  SaturateOnIntegerOverflow=off
  Product{,1..5} (6 alike) : Product
  Trigonometric Function : Trigonometry  Operator=cos
  Trigonometric Function1 : Trigonometry
  Trigonometric Function2 : Trigonometry  Operator=cos
  Trigonometric Function3 : Trigonometry
  Trigonometric Function4 : Trigonometry  Operator=cos
  Trigonometric Function5 : Trigonometry
  Duty Cycle A : Outport
  Duty Cycle A1 : Outport  Port=2
  Duty Cycle A2 : Outport  Port=3
  wires:
  Iq/1 -> [Id]  "d"
  Vq/1 -> [Iq]  "q"
  Add/1 -> Duty Cycle A/1  "a"
  Add1/1 -> Duty Cycle A1/1  "b"
  In3/1 -> [Theta]  "Theta"
  [Theta] -> Trigonometric Function1/1, Trigonometric Function/1
  [Iq] -> Product1/2
  Trigonometric Function/1 -> Product/2
  [Id] -> Product/1
  Trigonometric Function1/1 -> Product1/1
  Product/1 -> Add/1
  Product1/1 -> Add/2
  Product3/1 -> Add1/2
  [Theta] -> Bias/1
  [Id] -> Product2/1
  Product2/1 -> Add1/1
  Trigonometric Function3/1 -> Product3/1
  [Iq] -> Product3/2
  Trigonometric Function2/1 -> Product2/2
  Bias/1 -> Trigonometric Function3/1, Trigonometric Function2/1
  Trigonometric Function4/1 -> Product4/2
  [Id] -> Product4/1
  [Theta] -> Bias1/1
  [Iq] -> Product5/2
  Add2/1 -> Duty Cycle A2/1  "c"
  Product5/1 -> Add2/2
  Trigonometric Function5/1 -> Product5/1
  Product4/1 -> Add2/1
  Bias1/1 -> Trigonometric Function5/1, Trigonometric Function4/1

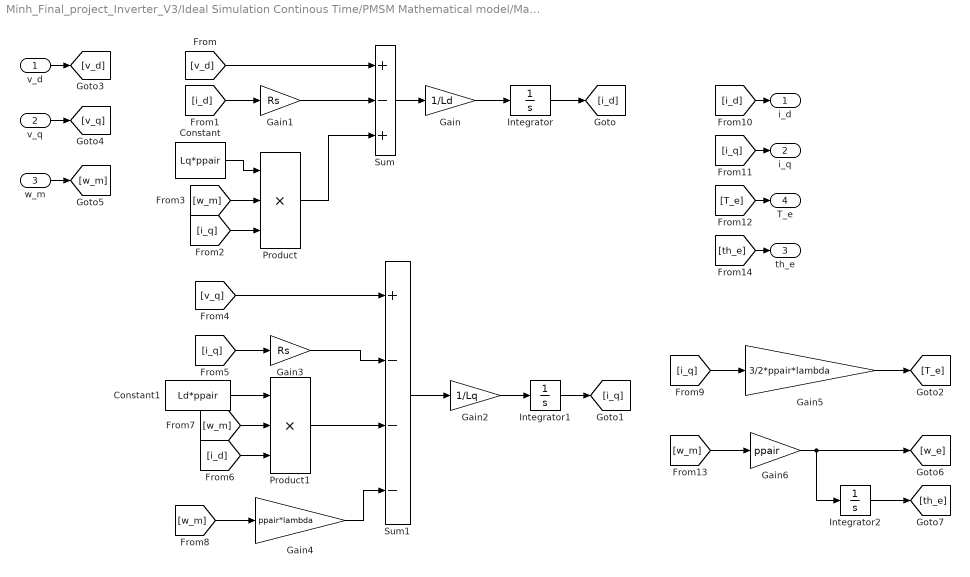
== system Minh_Final_project_Inverter_V3/Ideal Simulation Continous Time/PMSM Mathematical model/Machine Model in DQ ==
  v_d : Inport
  v_q : Inport  Port=2
  w_m : Inport  Port=3
  Constant : Constant  Value=Lq*ppair
  Constant1 : Constant  Value=Ld*ppair
  Gain : Gain  Gain=1/Ld
  Gain1 : Gain  Gain=Rs
  Gain2 : Gain  Gain=1/Lq
  Gain3 : Gain  Gain=Rs
  Gain4 : Gain  Gain=ppair*lambda
  Gain5 : Gain  Gain=3/2*ppair*lambda
  Gain6 : Gain  Gain=ppair
  Integrator : Integrator
  Integrator1 : Integrator
  Integrator2 : Integrator
  Product : Product  Inputs=3
  Product1 : Product  Inputs=3
  Sum : Sum  Inputs=+-+
  Sum1 : Sum  Inputs=+---
  i_d : Outport
  i_q : Outport  Port=2
  th_e : Outport  Port=3
  T_e : Outport  Port=4
  wires:
  Constant/1 -> Product/1
  Product/1 -> Sum/3
  Integrator/1 -> [i_d]
  [v_d] -> Sum/1
  [w_m] -> Product1/2
  Gain4/1 -> Sum1/4
  [i_q] -> Product/3
  Sum/1 -> Gain/1
  [w_m] -> Gain4/1
  [i_d] -> Gain1/1
  Sum1/1 -> Gain2/1
  Gain/1 -> Integrator/1
  Gain5/1 -> [T_e]
  [i_q] -> Gain5/1
  Gain1/1 -> Sum/2
  Integrator1/1 -> [i_q]
  [i_q] -> Gain3/1
  Product1/1 -> Sum1/3
  Constant1/1 -> Product1/1
  Gain2/1 -> Integrator1/1
  [v_q] -> Sum1/1
  Gain3/1 -> Sum1/2
  [i_d] -> Product1/3
  [w_m] -> Product/2
  v_d/1 -> [v_d]
  v_q/1 -> [v_q]
  [i_d] -> i_d/1
  [i_q] -> i_q/1
  [T_e] -> T_e/1
  w_m/1 -> [w_m]
  [w_m] -> Gain6/1
  Gain6/1 -> Integrator2/1, [w_e]
  Integrator2/1 -> [th_e]
  [th_e] -> th_e/1

== system Minh_Final_project_Inverter_V3/Ideal Simulation Continous Time/PMSM Mathematical model/Mechanical Model ==
  T_e : Inport
  Constant1 : Constant  Value=1/2*rho*C_d*A_f*r^2
  Constant2 : Constant  Value=m*g*C_rr
  Gain : Gain  Gain=1/k^2
  Product : Product
  Product2 : Product
  Sign : Signum
  Square : Math  Operator=square
  Subtract : Sum  Inputs=|+-
  Sum1 : Sum  Inputs=|++
  Transfer Fcn : TransferFcn  Denominator=[J 0]
  w_m : Outport
  wires:
  Constant1/1 -> Product2/1
  Transfer Fcn/1 -> Sign/1, Square/1, w_m/1
  Product2/1 -> Gain/1
  Square/1 -> Product2/2
  Subtract/1 -> Transfer Fcn/1
  T_e/1 -> Subtract/1
  Sum1/1 -> Subtract/2
  Gain/1 -> Sum1/1
  Constant2/1 -> Product/1
  Sign/1 -> Product/2
  Product/1 -> Sum1/2

== system Minh_Final_project_Inverter_V3/Ideal Simulation Continous Time/PWM and PMSM Simscape (real model)/Gate Driver ==
  Signal : Inport
  Constant2 : Constant
  Demux3 : Demux  Outputs=3
  Demux4 : Demux  Outputs=3
  Gain2 : Gain  Gain=12
  Gain3 : Gain  Gain=12
  Scope : Scope  NumInputPorts=2
  Simulink-PS Converter{3..8} (6 alike) : nesl_utility/Simulink-PS Converter  PhysicalDomain=network_engine_domain  SubClassName=ps_input  LeftPortType=input  RightPortType=output  PseudoPeriodic=off  Frequencies=[]  NoiseDistribution=none  NoiseParameters=[]  Unit=1  AffineConversion=off  FilteringAndDerivatives=provide  SimscapeFilterOrder=1  InputFilterTimeConstant=0.001  UdotUserProvided=0
  Six-Pulse Gate Multiplexer : ee_lib/Semiconductors & Converters/Converters/Six-Pulse Gate Multiplexer  port_option=ee.enum.controlport.ps
  Subtract6 : Sum  Inputs=|+-
  Gate : PMIOPort  Side=Right
  wires:
  Subtract6/1 -> Gain2/1
  Demux3/2 -> Simulink-PS Converter6/1
  Demux4/1 -> Scope/2, Simulink-PS Converter3/1
  Gain3/1 -> Demux4/1
  Demux3/3 -> Simulink-PS Converter8/1
  Demux4/3 -> Simulink-PS Converter7/1
  Signal/1 -> Gain3/1, Subtract6/2
  Demux4/2 -> Simulink-PS Converter5/1
  Gain2/1 -> Demux3/1
  Constant2/1 -> Subtract6/1
  Demux3/1 -> Scope/1, Simulink-PS Converter4/1
  connections:
  Simulink-PS Converter8/RConn1 -- Six-Pulse Gate Multiplexer/LConn6
  Simulink-PS Converter4/RConn1 -- Six-Pulse Gate Multiplexer/LConn2
  Simulink-PS Converter7/RConn1 -- Six-Pulse Gate Multiplexer/LConn5
  Simulink-PS Converter5/RConn1 -- Six-Pulse Gate Multiplexer/LConn3
  Simulink-PS Converter3/RConn1 -- Six-Pulse Gate Multiplexer/LConn1
  Simulink-PS Converter6/RConn1 -- Six-Pulse Gate Multiplexer/LConn4
  Six-Pulse Gate Multiplexer/RConn1 -- Gate/RConn1
